simulink library "simulink_need_slupdate"  (Simulink 7.1)
undefined symbols (not defined in the file or in its folder): Floor, getdatatypespecs
settings Model: Creator=dyang  LastModifiedBy=schim  ExtModeAutoUpdateStatusClock=off

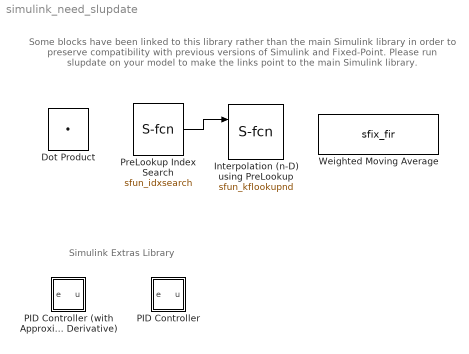
== system simulink_need_slupdate ==
  note: Some blocks have been linked to this library rather than the
      | main Simulink library in order to preserve compatibility with
      | previous versions of Simulink and Fixed-Point. Please run
      | slupdate on your model to make the links point to the main
      | Simulink library.
  note: Simulink Extras Library
  Dot Product : DotProduct  OutDataType=fixdt(1,16,2^0,0)  OutDataTypeStr=fixdt(1,16,2^0,0)
  Interpolation (n-D) using PreLookup : S-Function  FunctionName=sfun_kflookupnd  Parameters=numDims,table,interpMethod,extrapMethod,rangeErrorMode,NumSelectionDims  EnableBusSupport=off  mask(LookupNDInterpIdx){numDimsPopupSelect=2, explicitNumDims=2, table=sqrt([1:10]'*[1:10]), interpMethod=Linear, extrapMethod=Linear, rangeErrorMode=None, NumSelectionDims=0}
      mask prompts: numDimsPopupSelect "Number of table dimensions:"; explicitNumDims "Explicit number of table dimensions:"; table "Table data:"; interpMethod "Interpolation method:"; extrapMethod "Extrapolation method:"; rangeErrorMode "Action for out of range input:"; NumSelectionDims "Number of sub-table selection dimensions:"
      mask help: Perform interpolation on an n-dimensional (n-D) table using precalculated indices and distance fractions. An n-D Table is a sampled representation of a function in N variables. This block's 'u' input ports are intended to be fed with the output of a PreLook-Up Index Search block. Interpolation on a selected portion of the table can be optionally performed by specifying how many dimensions are to be used for sub-table selection. Sub-table selection is performed starting with the highest (last) dimension. The 'sel' input ports are fed with a uint32-typed value that is a table index in the corresponding dimension (zero-based indexing). The first dimension input corresponds to the top (or left) input port.
      mask init:
      | if numDimsPopupSelect==5
      |   numDims=explicitNumDims;
      | else
      |   numDims=numDimsPopupSelect;
      | end
      | [x,y,xaxes,yaxes] = ndlookico('plot',numDims, 'LookupNDInterpIdx', table, interpMethod, NumSelectionDims);
      mask StyleString: popup(1|2|3|4|More...),edit,edit,popup(None - Flat|Linear),popup(None - Clip|Linear),popup(None|Warning|Error|Error - No index checking in generated code|Warning - No index checking in generated code|None - No index checking in generated code),edit
      mask CallbackString: ndlookico('kfdyn')||||||
      mask Display:
      | text(0.5,0.9,' n-D T(k,f)','horizontalAlignment','center');
      | plot(x,y);
      | plot(xaxes,yaxes);
  PID Controller : Subsystem  mask(PID Controller){P=1, I=1, D=0}
      mask prompts: P "Proportional:"; I "Integral:"; D "Derivative:"
      mask help:
      | Enter expressions for proportional, integral, and derivative terms.
      | P+I/s+Ds
      mask Help: This block implements a PID controller where parameters are entered for the Proportional, Integral and Derivative terms. Unmask this block to see how it works. The derivative term is implemented using a true derivative block.
      mask Display: disp('PID')
  PID Controller (with Approximate Derivative) : Subsystem  mask(PID(2) Controller){P=1, I=1, D=0, N=100}
      mask prompts: P "Proportional:"; I "Integral:"; D "Derivative:"; N "Derivative divisor(N):"
      mask help:
      | Enter Proportional(P), Integral(I), and Derivative(D) and divisor (N) terms.
      | P+I/s+Ds/(1/Ns+1)
      mask Help: This block implements a PID controller where parameters are entered for the Proportional, Integral and Derivative and divisor terms. Unmask this block to see how it works. The derivative term is implemented using an s/(s/N +1)  transfer function block. Making N large can create a "stiff" system.
      mask Display: disp('PID')
  PreLookup Index Search : S-Function  FunctionName=sfun_idxsearch  Parameters=bpData, searchMode, cacheBpFlag, extrapMode, rangeErrorMode, outputFlag, IndexDataType  EnableBusSupport=off  mask(LookupIdxSearch){bpData=[10:10:100], searchMode=Binary Search, cacheBpFlag=off, outputFlag=off, IndexDataType=uint32, extrapMode=Linear Extrapolation, rangeErrorMode=None}
      mask prompts: bpData "Breakpoint data:"; searchMode "Index search method:"; cacheBpFlag "Begin index search using previous index result"; outputFlag "Output only the index"; IndexDataType "Index data type:"; extrapMode "Process out of range input:"; rangeErrorMode "Action for out of range input:"
      mask help: Locate the input value's relative position within a range of numbers (the "breakpoint data" set). Returns an array of the interval index "k"and distance fraction "f" that the input "u" reaches into the kth interval.
      mask init:
      | if outputFlag == 0
      |   fig = 'f';
      |   f = 'f';
      | else
      |   fig = 'k';
      |   f = '';
      | end
      | [x,y] = ndlookico('bpplotdata', fig);
      | [xp,yp] = ndlookico('bppatchdata');
      mask StyleString: edit,popup(Evenly Spaced Points|Linear Search|Binary Search),checkbox,checkbox,popup(uint32|int32),popup(Clip to Range|Linear Extrapolation),popup(None|Warning|Error)
      mask CallbackString: |||ndlookico('predyn')|||
      mask Display:
      | text(0.13, 0.85, 'u','HorizontalAlignment','center','VerticalAlignment','middle');
      | text(0.4, 0.53, ' k','HorizontalAlignment','center','VerticalAlignment','base');
      | text(0.88, 0.3, f,'HorizontalAlignment','center','VerticalAlignment','middle');
      | plot(x,y);
      | patch(xp, yp);
  Weighted Moving Average : S-Function  FunctionName=sfix_fir  Parameters=(getdatatypespecs(OutDataType,OutScaling,DblOver,0)),[DoSatur RndMeth-1],DblOver,dolog,mgainval,(getdatatypespecs(GainDataType,GainScaling,DblOver,RadixGroup)),samptime,vinit,OutputDataTypeScalingMode,GainDataTypeScalingMode  EnableBusSupport=off  mask(Weighted Moving Average){mgainval=[0.1:0.1:1 0.9:-0.1:0.1], vinit=0.0, samptime=-1, OutDataTypeStr=Inherit: Inherit via internal rule, OutputDataTypeScalingMode=Inherit via internal rule, OutDataType=sfix(16), OutScaling=2^-10, LockScale=off, RndMeth=Floor, DoSatur=off, GainDataTypeStr=Inherit: Inherit via internal rule, GainDataTypeScalingMode=Inherit via internal rule, GainDataType=sfix( 16 ), MatRadixGroup=Best Precision: Matrix-wise, GainScaling=2^-10}
      mask prompts: mgainval "Weights:"; vinit "Initial condition:"; samptime "Sample time:"; OutDataTypeStr "Output data type:"; OutputDataTypeScalingMode "Output data type mode:"; OutDataType "Output data type (e.g. sfix(16), uint(8), float('single')):"; OutScaling "Output scaling (Slope, e.g. 2^-9 or [Slope Bias], e.g. [1.25 3]):"; LockScale "Lock output scaling against changes by the autoscaling tool"; RndMeth "Integer rounding mode:"; DoSatur "Saturate to max or min when overflows occur"; GainDataTypeStr "Gain data type:"; GainDataTypeScalingMode "Gain data type mode:"; GainDataType "Parameter data type (e.g. sfix(16), uint(8), float('single')):"; MatRadixGroup "Parameter scaling mode:"; GainScaling "Parameter scaling (Slope, e.g. 2^-9):"
      mask help: Output the weighted moving average of the input.
      mask init:
      | DblOver = 0;
      | dolog = 0;
      | 
      | switch MatRadixGroup
      | case 1
      |    RadixGroup = 0; % BEST_PREC_OFF
      | case 5
      |    RadixGroup = 1; % BEST_PREC_MAT
      | case {2,3,4};
      |    % Deprecate non-matrix best precision
      |    set_param(gcb, 'MatRadixGroup', 'Best Precision: Matrix-wise');
      | end
      mask StyleString: edit,edit,edit,unidt({m=4|5|6||7|||}{i=Inherit: Inherit via internal rule|Inherit: Inherit via back propagation}{s=UDTBinaryPointMode|UDTSlopeBiasMode}{g=UDTSignedSign|UDTUnsignedSign}),popup(Specify via dialog|Inherit via internal rule|Inherit via back propagation),edit,edit,checkbox,popup(Ceiling|Convergent|Floor|Nearest|Round|Simplest|Zero),checkbox,unidt({m=11|12|13|14|15|||1}{i=Inherit: Inherit via internal rule}{s=UDTBinaryPointMode|UDTSlopeBiasMode|UDTBestPrecisionMode}{g=UDTSignedSign|UDTUnsignedSign}),popup(Specify via dialog|Inherit via internal rule),edit,popup(Use specified scaling|Best Precision: Element-wise|Best Precision: Row-wise|Best Precision: Column-wise|Best Precision: Matrix-wise),edit
      mask CallbackString: |||fixptdialog(gcbh)|fixptdialog(gcbh)|fixptdialog(gcbh)|||||fixptdialog(gcbh)|fixptdialog(gcbh)|fixptdialog(gcbh)|fixptdialog(gcbh)|
      mask TabNameString: Main,Main,Main,Signal Attributes,Signal Attributes,Signal Attributes,Signal Attributes,Signal Attributes,Signal Attributes,Signal Attributes,Parameter Attributes,Parameter Attributes,Parameter Attributes,Parameter Attributes,Parameter Attributes
      mask Display:
      | fprintf(fixpt_fir_mask_data(mgainval,'dispstr'))
      | plot(fixpt_fir_mask_data(mgainval,1),fixpt_fir_mask_data(mgainval,0))
  wires:
  PreLookup Index Search/1 -> Interpolation (n-D) using PreLookup/1

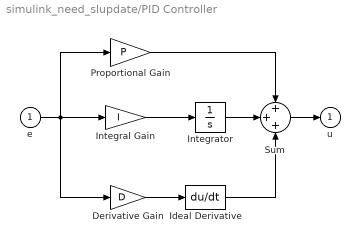
== system simulink_need_slupdate/PID Controller ==
  e : Inport  OutDataType=sfix(16)  OutScaling=2^0
  Derivative Gain : Gain  Gain=D  ParameterDataType=sfix(16)  ParameterScaling=2^0  OutDataType=sfix(16)  OutScaling=2^0
  Ideal Derivative : Derivative
  Integral Gain : Gain  Gain=I  ParameterDataType=sfix(16)  ParameterScaling=2^0  OutDataType=sfix(16)  OutScaling=2^0
  Integrator : Integrator
  Proportional Gain : Gain  Gain=P  ParameterDataType=sfix(16)  ParameterScaling=2^0  OutDataType=sfix(16)  OutScaling=2^0
  Sum : Sum  Inputs=+++  OutDataType=sfix(16)  OutScaling=2^0
  u : Outport  OutDataType=sfix(16)  OutScaling=2^0  InitialOutput=0
  wires:
  Derivative Gain/1 -> Ideal Derivative/1
  Sum/1 -> u/1
  e/1 -> Integral Gain/1, Proportional Gain/1, Derivative Gain/1
  Ideal Derivative/1 -> Sum/3
  Integrator/1 -> Sum/2
  Proportional Gain/1 -> Sum/1
  Integral Gain/1 -> Integrator/1

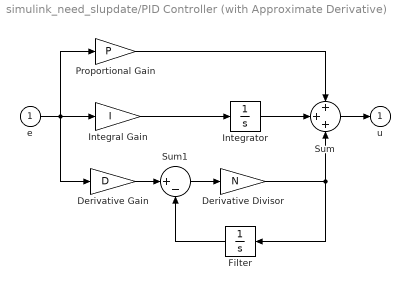
== system simulink_need_slupdate/PID Controller (with Approximate Derivative) ==
  e : Inport  OutDataType=sfix(16)  OutScaling=2^0
  Derivative Divisor : Gain  Gain=N  ParameterDataType=sfix(16)  ParameterScaling=2^0  OutDataType=sfix(16)  OutScaling=2^0
  Derivative Gain : Gain  Gain=D  ParameterDataType=sfix(16)  ParameterScaling=2^0  OutDataType=sfix(16)  OutScaling=2^0
  Filter : Integrator
  Integral Gain : Gain  Gain=I  ParameterDataType=sfix(16)  ParameterScaling=2^0  OutDataType=sfix(16)  OutScaling=2^0
  Integrator : Integrator
  Proportional Gain : Gain  Gain=P  ParameterDataType=sfix(16)  ParameterScaling=2^0  OutDataType=sfix(16)  OutScaling=2^0
  Sum : Sum  Inputs=+++  OutDataType=sfix(16)  OutScaling=2^0
  Sum1 : Sum  Inputs=|+-  OutDataType=sfix(16)  OutScaling=2^0
  u : Outport  OutDataType=sfix(16)  OutScaling=2^0  InitialOutput=0
  wires:
  Filter/1 -> Sum1/2
  Derivative Divisor/1 -> Sum/3, Filter/1
  Derivative Gain/1 -> Sum1/1
  Sum1/1 -> Derivative Divisor/1
  Integral Gain/1 -> Integrator/1
  Sum/1 -> u/1
  e/1 -> Proportional Gain/1, Integral Gain/1, Derivative Gain/1
  Integrator/1 -> Sum/2
  Proportional Gain/1 -> Sum/1
